simulink library "ControledSyncGenLib"  (R2013a)
settings: Solver=ode45  StartTime=0.0  StopTime=10.0  RelTol=1e-3
libraries: powerlib x5, powerlib_meascontrol x1, SyncGenLib x1
settings Model: Creator=USER  LastModifiedBy=USER

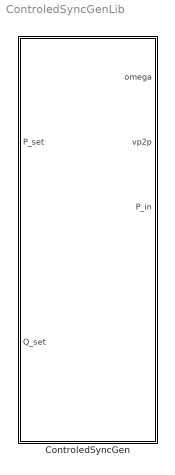
== system ControledSyncGenLib ==
  ControledSyncGen : Subsystem  mask{R_f=0.1, R_s=0.1, D_p=0.1, J=0.1, M_f=0.1, L_f=0.1, L_s=0.1, Omega_0=0, Theta_0=0, K_p=0.1, D_q=20, K=1}
      mask prompts: R_f "Value of the rotor resistor"; R_s "Value of the stator resistor"; D_p "The viscose frection droop factor"; J "Rotor momont of inertia"; M_f "The rotror-stator inductance factor"; L_f "The rotor inductance factor"; L_s "The stator inductance factor"
      mask TypeOptions R_f:
      | SyncGen
      | /R_f
      mask TypeOptions R_s:
      | SyncGen
      | /R_s
      mask TypeOptions D_p:
      | SyncGen
      | /D_p
      mask TypeOptions J:
      | SyncGen
      | /J
      mask TypeOptions M_f:
      | SyncGen
      | /M_f
      mask TypeOptions L_f:
      | SyncGen
      | /L_f
      mask TypeOptions L_s:
      | SyncGen
      | /L_s
      mask TypeOptions Omega_0:
      | SyncGen
      | /Omega_0
      mask TypeOptions Theta_0:
      | SyncGen
      | /Theta_0

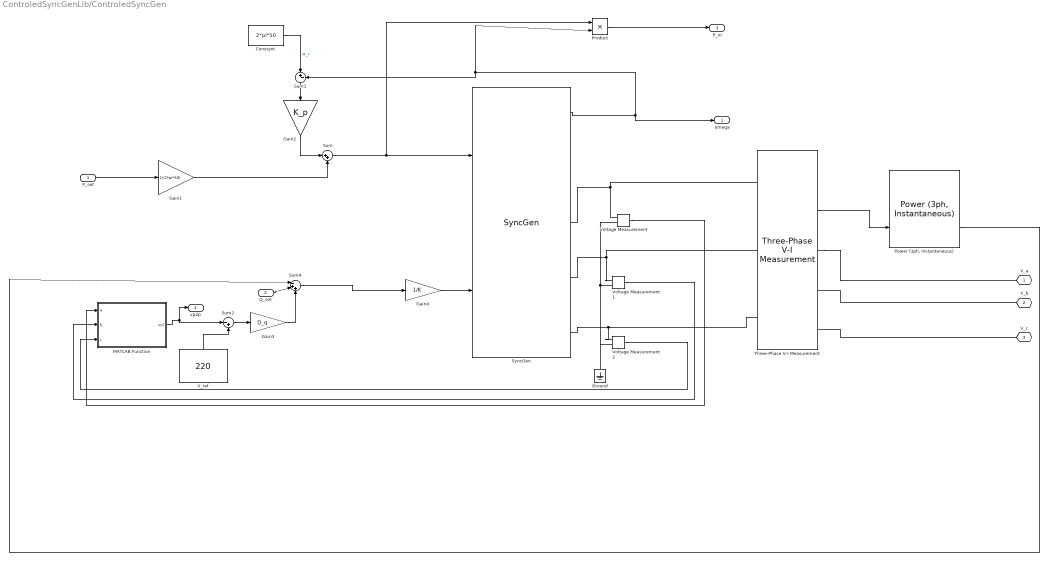
== system ControledSyncGenLib/ControledSyncGen ==
  "P_set " : Inport
  Q_set : Inport  Port=2
  Constant : Constant  Value=2*pi*50
  Gain1 : Gain  Gain=1/(2*pi*50)
  Gain2 : Gain  Gain=K_p
  Gain3 : Gain  Gain=D_q
  Gain4 : Gain  Gain=1/K
  Ground : powerlib/Elements/Ground  LConnTagsString=a
  MATLAB Function : MATLAB Function  TreatAsAtomicUnit=on
  "Power (3ph, Instantaneous)" : powerlib_meascontrol/Measurements/Power (3ph, Instantaneous)
  Product : Product
  Sum : Sum  Inputs=|++
  Sum1 : Sum  Inputs=|+-
  Sum2 : Sum  Inputs=|-+
  Sum4 : Sum  Inputs=|-++
  "SyncGen " : SyncGenLib/SyncGen   R_f=R_f  R_s=R_s  D_p=D_p  J=J  M_f=M_f  L_f=L_f  L_s=L_s  Omega_0=Omega_0  Theta_0=Theta_0
  Three-Phase V-I Measurement : powerlib/Measurements/Three-Phase V-I Measurement  VoltageMeasurement=phase-to-ground  SetLabelV=off  LabelV=Vabc  Vpu=off  VpuLL=off  CurrentMeasurement=yes  SetLabelI=off  LabelI=Iabc  Ipu=off  Pbase=100e6  Vbase=500e3  OutputType=Complex  PhasorSimulation=off  PSBequivalent=0
  V_ref : Constant  Value=220
  Voltage Measurement : powerlib/Measurements/Voltage Measurement  PhasorSimulation=off  OutputType=Complex  PSBequivalent=0
  Voltage Measurement1 : powerlib/Measurements/Voltage Measurement  PhasorSimulation=off  OutputType=Complex  PSBequivalent=0
  Voltage Measurement2 : powerlib/Measurements/Voltage Measurement  PhasorSimulation=off  OutputType=Complex  PSBequivalent=0
  V_a : PMIOPort  Tag=PMCPort  Port=1  Side=Right
  V_b : PMIOPort  Tag=PMCPort  Port=2  Side=Right
  V_c : PMIOPort  Tag=PMCPort  Port=3  Side=Right
  omega : Outport
  vp2p : Outport  Port=2
  P_in : Outport  Port=3
  wires:
  "SyncGen "/1 -> omega/1, Product/2, Sum1/2
  Sum1/1 -> Gain2/1
  Constant/1 -> Sum1/1  "w_r"
  Voltage Measurement/1 -> MATLAB Function/1(a)
  Voltage Measurement2/1 -> MATLAB Function/3(c)
  Voltage Measurement1/1 -> MATLAB Function/2(b)
  MATLAB Function/1(vol) -> vp2p/1, Sum2/1
  V_ref/1 -> Sum2/2
  Gain4/1 -> "SyncGen "/2
  Product/1 -> P_in/1
  "P_set "/1 -> Gain1/1
  Gain2/1 -> Sum/1
  Gain1/1 -> Sum/2
  Sum/1 -> Product/1, "SyncGen "/1
  Three-Phase V-I Measurement/2 -> "Power (3ph, Instantaneous)"/2
  Sum2/1 -> Gain3/1
  Gain3/1 -> Sum4/3
  "Power (3ph, Instantaneous)"/2 -> Sum4/1
  Q_set/1 -> Sum4/2
  Sum4/1 -> Gain4/1
  connections:
  Voltage Measurement/LConn1 -- Three-Phase V-I Measurement/LConn1 -- "SyncGen "/RConn1
  "SyncGen "/RConn3 -- Three-Phase V-I Measurement/LConn3 -- Voltage Measurement2/LConn1
  "SyncGen "/RConn2 -- Three-Phase V-I Measurement/LConn2 -- Voltage Measurement1/LConn1
  Voltage Measurement1/LConn2 -- Voltage Measurement/LConn2 -- Ground/LConn1 -- Voltage Measurement2/LConn2
  Three-Phase V-I Measurement/RConn1 -- V_a/RConn1
  V_b/RConn1 -- Three-Phase V-I Measurement/RConn2
  V_c/RConn1 -- Three-Phase V-I Measurement/RConn3

== matlab function ControledSyncGenLib/ControledSyncGen/MATLAB Function ==
  data: a input; vol output; b input; c input
function vol = P2PVoltageDetector(a,b,c)
vol = sqrt(a^2 + b^2 + c^2)*2/3;
